simulink model "Aearial_Inspection_UAV_Simulation"  (R2023a)
settings: Solver=daessc  StartTime=0.0  StopTime=tf  MaxStep=0.1  MinStep=1e-30  RelTol=1e-4
values from neighbouring files (symbols this model uses):
  arm_start = 0    [InitScript.m]
  X = T*[x0;y0]    [line2circle.m]
undefined symbols (not defined in the file or in its folder): arm_end, DiscIntNeverNeededParam, F, is_gust_active, Light, MIL, Mode, Motor_data, params, Robotic_Arm_ASM_DataFile, Sensor_err, servo_specs, simple_env, stepper, Tm, wind_speed, xStack1, xStack2, Y, Z
libraries: sm_lib x399, nesl_utility x78, simulink x25, dspsrcs4 x16, simulink_extras x8, sharedtransform x7, aerolibwind2 x2, sharedutil x1
(part 2 of 12)

== system Aearial_Inspection_UAV_Simulation/UAV/Flange 1-1 ==
  PS-Simulink Converter : nesl_utility/PS-Simulink Converter  PhysicalDomain=network_engine_domain  SubClassName=ps_output  LeftPortType=input  RightPortType=output  PseudoPeriodic=off  Frequencies=[]  VectorFormat=1-D array  Unit=deg  AffineConversion=off
  Revolute : sm_lib/Joints/Revolute Joint  JointMode=Normal  SenseConstraintForce=off  SenseConstraintForceX=off  SenseConstraintForceY=off  SenseConstraintForceZ=off  SenseConstraintTorque=off  SenseConstraintTorqueX=off  SenseConstraintTorqueY=off  SenseConstraintTorqueZ=off  SenseTotalForce=off  SenseTotalForceX=off  SenseTotalForceY=off  SenseTotalForceZ=off  SenseTotalTorque=off  SenseTotalTorqueX=off  SenseTotalTorqueY=off  SenseTotalTorqueZ=off  CompositeWrenchDir=FollowerOnBase  CompositeWrenchFrame=BaseFrame  EquilibriumPosition=-360*2  EquilibriumPositionUnits=deg  SpringStiffness=1e-5  SpringStiffnessUnits=N*m/deg  DampingCoefficient=3e-6  DampingCoefficientUnits=N*m/(deg/s)  TorqueActuationMode=NoTorque  MotionActuationMode=ComputedMotion  SensePosition=on  SenseVelocity=off  SenseAcceleration=off  SenseTorqueForce=off  SenseLowerLimitTorqueForce=off  SenseUpperLimitTorqueForce=off  LowerLimitSpecify=on  LowerLimitBound=0  LowerLimitBoundUnits=deg  LowerLimitStiffness=1e-2  LowerLimitStiffnessUnits=N*m/deg  LowerLimitDamping=1  LowerLimitDampingUnits=N*m/(deg/s)  LowerLimitTransitionRegionWidth=0.1  LowerLimitTransitionRegionWidthUnits=deg  UpperLimitSpecify=on  UpperLimitBound=80  UpperLimitBoundUnits=deg  UpperLimitStiffness=1  UpperLimitStiffnessUnits=N*m/deg  UpperLimitDamping=1000  UpperLimitDampingUnits=N*m/(deg/s)  UpperLimitTransitionRegionWidth=0.1  UpperLimitTransitionRegionWidthUnits=deg  PositionTargetSpecify=on  PositionTargetPriority=Low  PositionTargetValue=10  PositionTargetValueUnits=deg  VelocityTargetSpecify=off  VelocityTargetPriority=High  VelocityTargetValue=0  VelocityTargetValueUnits=deg/s
  Transform : sm_lib/Frames and Transforms/Rigid Transform  TranslationMethod=Cartesian  TranslationStandardOffset=0  TranslationStandardOffsetUnits=m  TranslationStandardAxis=+Z  TranslationCartesianOffset=env.flange1_1.pos  TranslationCartesianOffsetUnits=m  TranslationROffset=0  TranslationROffsetUnits=m  TranslationZOffset=0  TranslationZOffsetUnits=m  TranslationThetaOffset=0  TranslationThetaOffsetUnits=deg  RotationMethod=RotationSequence  RotationAngleUnits=rad  RotationStandardAxis=+Z  RotationAngle=smiData.RigidTransform(3).angle  RotationArbitraryAxis=smiData.RigidTransform(3).axis  FollAlignAxisA=+X  BaseAlignAxisA=+Y  FollAlignAxisB=+Y  BaseAlignAxisB=+Z  RotationSequenceAxes=BaseAxes  RotationSequence=ZYX  RotationSequenceAngles=[90 -90 0]  RotationSequenceAnglesUnits=deg  RotationMatrix=[1 0 0; 0 1 0; 0 0 1]  Quaternion=[1 0 0 0]
  flange_1_RIGID : Subsystem
  flange_gate_1_RIGID : Subsystem
  Conn1 : PMIOPort  Side=Left
  Flange Door : PMIOPort  Port=2  Side=Right
  rot flange 1-1 : Outport
  wires:
  PS-Simulink Converter/1 -> rot flange 1-1/1
  connections:
  Conn1/RConn1 -- Transform/LConn1
  Transform/RConn1 -- flange_1_RIGID/LConn1
  Revolute/RConn1 -- flange_gate_1_RIGID/LConn1
  Revolute/LConn1 -- flange_1_RIGID/RConn1
  Flange Door/RConn1 -- flange_gate_1_RIGID/LConn2
  Revolute/RConn2 -- PS-Simulink Converter/LConn1

== system Aearial_Inspection_UAV_Simulation/UAV/Robotic Arm ==
  servos pos [6] : Inport
  Degrees to Radians : simulink_extras/Transformations/Degrees to Radians
  Demux : Demux  Outputs=6
  Gain : Gain  Gain=-1
  Gain2 : Gain  Gain=-1
  Mux : Mux  Inputs=6
  Robotic Arm and Servos : Subsystem
  Transport Delay : TransportDelay  DelayTime=0.001
  Transport Delay1 : TransportDelay  DelayTime=0.001
  ArmHolder : PMIOPort  Side=Left
  prob Geo : PMIOPort  Port=2  Side=Left
  prob head : PMIOPort  Port=3  Side=Left
  arms_real_rot_deg : Outport
  probHeadPos (disconnected) : Outport  Port=2
  probDiskPos : Outport  Port=3
  wires:
  Demux/5 -> Gain2/1
  Demux/6 -> Robotic Arm and Servos/6(w3)
  Transport Delay1/1 -> probDiskPos/1
  Degrees to Radians/1 -> Demux/1
  Transport Delay/1 -> arms_real_rot_deg/1
  Gain/1 -> Robotic Arm and Servos/1(a0)
  Robotic Arm and Servos/8(probDiskPos) -> Transport Delay1/1
  Robotic Arm and Servos/7(probHeadPos (disconnected)) -> probHeadPos (disconnected)/1
  Robotic Arm and Servos/6(w3_real) -> Mux/6
  Robotic Arm and Servos/4(w1_real) -> Mux/4
  Robotic Arm and Servos/5(w2_real) -> Mux/5
  Robotic Arm and Servos/2(a1_real) -> Mux/2
  Robotic Arm and Servos/3(a2_real) -> Mux/3
  Robotic Arm and Servos/1(a0_real) -> Mux/1
  Mux/1 -> Transport Delay/1
  servos pos [6]/1 -> Degrees to Radians/1
  Demux/4 -> Robotic Arm and Servos/4(w1)
  Gain2/1 -> Robotic Arm and Servos/5(w2)
  Demux/3 -> Robotic Arm and Servos/3(a2)
  Demux/1 -> Gain/1
  Demux/2 -> Robotic Arm and Servos/2(a1)
  connections:
  prob head/RConn1 -- Robotic Arm and Servos/LConn3
  prob Geo/RConn1 -- Robotic Arm and Servos/LConn2
  ArmHolder/RConn1 -- Robotic Arm and Servos/LConn1

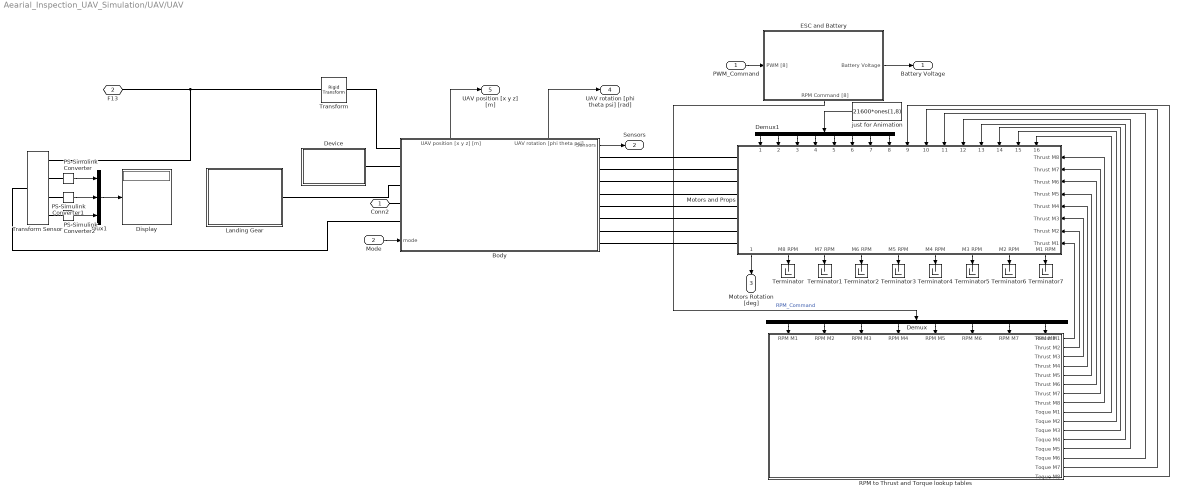
== system Aearial_Inspection_UAV_Simulation/UAV/UAV ==
  PWM_Command : Inport
  Mode : Inport  Port=2
  Body : Subsystem
      settings: PortSchema="{\"entries\":[{\"content\":{\"sides\":[{\"content\":{\"connectorIds\":[\"LConn1\",\"LConn2\",\"LConn3\",\"LConn4\",\"LConn5\",\"In1\"]},\"type\":\"ConnectorPlacement.EquallySpacedRectSide\",\"uuid\":\"8abbfab2-f266-443b-993d-92a00d5129d3\"},{\"content\":{\"connectorIds\":[\"Out1\",\"RConn1\",\"RConn2\",\"RConn3\",\"RConn4\",\"RConn5\",\"RConn6\",\"RConn7\",\"RConn8\"],\"side\":\"RIGHT\"},\"type\":\"ConnectorPlacement.EquallySpacedRectSide\",\"uuid\":\"d3862e7a-1f62-4fff-84ef-3f151d54fb23\"},{\"content\":{\"connectorIds\":[\"Out2\",\"Out3\"],\"side\":\"TOP\"},\"type\":\"ConnectorPlacement.EquallySpacedRectSide\",\"uuid\":\"186dc438-5235-44e9-8ffb-2a07ea9e8cef\"}]},\"type\":\"ConnectorPlacement.EquallySpacedConnector\",\"uuid\":\"6424af0a-0cb2-4ac3-b98a-3d9cf8166d6d\"}],\"packageUris\":[\"http://schema.mathworks.com/mf0/Connector/R2020b\"],\"version\":\"1.0\"}"
      mask Display: image('D:\MS_Control_Project\pictures\CH5\UAV.JPG'); % Use "Edit Image" on toolstrip to change.
  Demux : Demux  Outputs=8
  Demux1 : Demux  Outputs=8
  Device : Subsystem
      mask Display: image('D:\MS_Control_Project\pictures\CH3\test350.JPG'); % Use "Edit Image" on toolstrip to change.
  Display : Display
  ESC and Battery : Subsystem
      settings: PortSchema="{\"entries\":[{\"content\":{\"sides\":[{\"content\":{\"connectorIds\":[]},\"type\":\"ConnectorPlacement.EquallySpacedRectSide\",\"uuid\":\"711663de-8dcc-49e0-b3a9-e528dcc5693d\"},{\"content\":{\"connectorIds\":[\"Out1\"],\"side\":\"RIGHT\"},\"type\":\"ConnectorPlacement.EquallySpacedRectSide\",\"uuid\":\"6f86bd31-ad4a-448e-be8f-fb164a73c091\"},{\"content\":{\"connectorIds\":[\"In1\"],\"side\":\"TOP\"},\"type\":\"ConnectorPlacement.EquallySpacedRectSide\",\"uuid\":\"20362943-c19a-4854-b367-6ab35e814521\"},{\"content\":{\"connectorIds\":[\"Out2\"],\"side\":\"BOTTOM\"},\"type\":\"ConnectorPlacement.EquallySpacedRectSide\",\"uuid\":\"05de8953-dfce-4a54-9043-b5e6de62a3cd\"}]},\"type\":\"ConnectorPlacement.EquallySpacedConnector\",\"uuid\":\"7185b2e0-7de4-4151-8ca9-e57776bd11c7\"}],\"packageUris\":[\"http://schema.mathworks.com/mf0/Connector/R2020b\"],\"version\":\"1.0\"}"
  Landing Gear : Subsystem
  Motors and Props : Subsystem
      settings: PortSchema="{\"entries\":[{\"content\":{\"sides\":[{\"content\":{\"connectorIds\":[\"LConn1\",\"LConn2\",\"LConn3\",\"LConn4\",\"LConn5\",\"LConn6\",\"LConn7\",\"LConn8\"]},\"type\":\"ConnectorPlacement.EquallySpacedRectSide\",\"uuid\":\"df44c6ad-f38c-4e0a-a4d8-2c23b112f28a\"},{\"content\":{\"connectorIds\":[\"In17\",\"In18\",\"In19\",\"In20\",\"In21\",\"In22\",\"In23\",\"In24\"],\"side\":\"RIGHT\"},\"type\":\"ConnectorPlacement.EquallySpacedRectSide\",\"uuid\":\"523caf36-7a83-48a0-a73d-1fb2051ba00a\"},{\"content\":{\"connectorIds\":[\"In1\",\"In2\",\"In3\",\"In4\",\"In5\",\"In6\",\"In7\",\"In8\",\"In9\",\"In10\",\"In11\",\"In12\",\"In13\",\"In14\",\"In15\",\"In16\"],\"side\":\"TOP\"},\"type\":\"ConnectorPlacement.EquallySpacedRectSide\",\"uuid\":\"ed00d928-f4f1-4152-a592-487d88c7be46\"},{\"content\":{\"connectorIds\":[\"Out1\",\"Out2\",\"Out3\",\"Out4\",\"Out5\",\"Out6\",\"Out7\",\"Out8\",\"Out9\"],\"side\":\"BOTTOM\"},\"type\":\"ConnectorPlacement.EquallySpacedRectSide\",\"uuid\":\"181016b2-11c7-4594-b58c-8221d4cffb47\"}]},\"type\":\"ConnectorPlacement.EquallySpacedConnector\",\"uuid\":\"b878f0ff-a82a-4258-9edd-ea8bbdd36818\"}],\"packageUris\":[\"http://schema.mathworks.com/mf0/Connector/R2020b\"],\"version\":\"1.0\"}"
      mask Display: image('D:\MS_Control_Project\pictures\CH3\p60 with prop.JPG'); % Use "Edit Image" on toolstrip to change.
  Mux1 : Mux  Inputs=3
  PS-Simulink Converter : nesl_utility/PS-Simulink Converter  PhysicalDomain=network_engine_domain  SubClassName=ps_output  LeftPortType=input  RightPortType=output  PseudoPeriodic=off  Frequencies=[]  VectorFormat=1-D array  Unit=inherit  AffineConversion=off
  PS-Simulink Converter1 : nesl_utility/PS-Simulink Converter  PhysicalDomain=network_engine_domain  SubClassName=ps_output  LeftPortType=input  RightPortType=output  PseudoPeriodic=off  Frequencies=[]  VectorFormat=1-D array  Unit=inherit  AffineConversion=off
  PS-Simulink Converter2 : nesl_utility/PS-Simulink Converter  PhysicalDomain=network_engine_domain  SubClassName=ps_output  LeftPortType=input  RightPortType=output  PseudoPeriodic=off  Frequencies=[]  VectorFormat=1-D array  Unit=inherit  AffineConversion=off
  RPM to Thrust and Torque lookup tables : Subsystem
      settings: PortSchema="{\"entries\":[{\"content\":{\"sides\":[{\"content\":{\"connectorIds\":[]},\"type\":\"ConnectorPlacement.EquallySpacedRectSide\",\"uuid\":\"e225c0ad-404f-4beb-bd3c-0cf073c7c3b6\"},{\"content\":{\"connectorIds\":[\"Out1\",\"Out2\",\"Out3\",\"Out4\",\"Out5\",\"Out6\",\"Out7\",\"Out8\",\"Out9\",\"Out10\",\"Out11\",\"Out12\",\"Out13\",\"Out14\",\"Out15\",\"Out16\"],\"side\":\"RIGHT\"},\"type\":\"ConnectorPlacement.EquallySpacedRectSide\",\"uuid\":\"ade02e52-3795-4ae7-8485-9b36c688ef9f\"},{\"content\":{\"connectorIds\":[\"In1\",\"In2\",\"In3\",\"In4\",\"In5\",\"In6\",\"In7\",\"In8\"],\"side\":\"TOP\"},\"type\":\"ConnectorPlacement.EquallySpacedRectSide\",\"uuid\":\"a41127fa-8705-473b-8191-192aa5d830a9\"}]},\"type\":\"ConnectorPlacement.EquallySpacedConnector\",\"uuid\":\"d5038a5f-1241-42ee-bed9-472ac5262e65\"}],\"packageUris\":[\"http://schema.mathworks.com/mf0/Connector/R2020b\"],\"version\":\"1.0\"}"
  Terminator{,1..7} (8 alike) : Terminator
  Transform : sm_lib/Frames and Transforms/Rigid Transform  TranslationMethod=Cartesian  TranslationStandardOffset=0  TranslationStandardOffsetUnits=mm  TranslationStandardAxis=+Z  TranslationCartesianOffset=[-138 23.5 29.5]  TranslationCartesianOffsetUnits=mm  TranslationROffset=0  TranslationROffsetUnits=m  TranslationZOffset=0  TranslationZOffsetUnits=m  TranslationThetaOffset=0  TranslationThetaOffsetUnits=deg  RotationMethod=StandardAxis  RotationAngleUnits=deg  RotationStandardAxis=+Z  RotationAngle=-90  RotationArbitraryAxis=smiData.RigidTransform(37).axis  FollAlignAxisA=+X  BaseAlignAxisA=+Y  FollAlignAxisB=+Y  BaseAlignAxisB=+Z  RotationSequenceAxes=FollowerAxes  RotationSequence=XYX  RotationSequenceAngles=[0 0 0]  RotationSequenceAnglesUnits=deg  RotationMatrix=[1 0 0; 0 1 0; 0 0 1]  Quaternion=[1 0 0 0]
  Transform Sensor : sm_lib/Frames and Transforms/Transform Sensor  MeasurementFrame=Base  RotationSequence=XYX  SenseAngle=off  SenseAxis=off  SenseQ=off  SenseR=off  SenseRotationSequence=off  SenseOmegaX=off  SenseOmegaY=off  SenseOmegaZ=off  SenseQDot=off  SenseRDot=off  SenseRotationSequenceDot=off  SenseAlphaX=off  SenseAlphaY=off  SenseAlphaZ=off  SenseQDDot=off  SenseRDDot=off  SenseX=on  SenseY=on  SenseZ=on  SenseRad=off  SenseAzim=off  SenseDist=off  SenseInc=off  SenseXDot=off  SenseYDot=off  SenseZDot=off  SenseRadDot=off  SenseAzimDot=off  SenseDistDot=off  SenseIncDot=off  SenseXDDot=off  SenseYDDot=off  SenseZDDot=off  SenseRadDDot=off  SenseAzimDDot=off  SenseDistDDot=off  SenseIncDDot=off
  just for Animation : Constant  Value=21600*ones(1,8)
  Conn2 : PMIOPort  Side=Left
  F13 : PMIOPort  Port=2  Side=Left
  Battery Voltage : Outport
  Sensors : Outport  Port=2
  Motors Rotation [deg] : Outport  Port=3
  UAV rotation [phi theta psi] [rad] : Outport  Port=4
  UAV position [x y z] [m] : Outport  Port=5
  wires:
  PWM_Command/1 -> ESC and Battery/1(PWM [8])
  ESC and Battery/1(RPM Command [8]) -> Demux/1  "RPM_Command"
  RPM to Thrust and Torque lookup tables/1(Thrust M1) -> Motors and Props/24(Thrust M1)
  RPM to Thrust and Torque lookup tables/2(Thrust M2) -> Motors and Props/23(Thrust M2)
  RPM to Thrust and Torque lookup tables/3(Thrust M3) -> Motors and Props/22(Thrust M3)
  RPM to Thrust and Torque lookup tables/4(Thrust M4) -> Motors and Props/21(Thrust M4)
  RPM to Thrust and Torque lookup tables/5(Thrust M5) -> Motors and Props/20(Thrust M5)
  RPM to Thrust and Torque lookup tables/6(Thrust M6) -> Motors and Props/19(Thrust M6)
  RPM to Thrust and Torque lookup tables/7(Thrust M7) -> Motors and Props/18(Thrust M7)
  RPM to Thrust and Torque lookup tables/8(Thrust M8) -> Motors and Props/17(Thrust M8)
  RPM to Thrust and Torque lookup tables/9(Toque M1) -> Motors and Props/16(Torque M1)
  RPM to Thrust and Torque lookup tables/10(Toque M2) -> Motors and Props/15(Torque M2)
  RPM to Thrust and Torque lookup tables/11(Toque M3) -> Motors and Props/14(Torque M3)
  RPM to Thrust and Torque lookup tables/12(Toque M4) -> Motors and Props/13(Torque M4)
  RPM to Thrust and Torque lookup tables/13(Toque M5) -> Motors and Props/12(Torque M5)
  RPM to Thrust and Torque lookup tables/14(Toque M6) -> Motors and Props/11(Torque M6)
  RPM to Thrust and Torque lookup tables/15(Toque M7) -> Motors and Props/10(Torque M7)
  RPM to Thrust and Torque lookup tables/16(Toque M8) -> Motors and Props/9(Torque M8)
  ESC and Battery/2(Battery Voltage) -> Battery Voltage/1
  Body/1(Sensors) -> Sensors/1
  Motors and Props/1(Motors Rotation [deg]) -> Motors Rotation [deg]/1
  Body/3(UAV rotation [phi theta psi]) -> UAV rotation [phi theta psi] [rad]/1
  Body/2(UAV position [x y z] [m]) -> UAV position [x y z] [m]/1
  Demux/8 -> RPM to Thrust and Torque lookup tables/8(RPM M8)
  Demux/7 -> RPM to Thrust and Torque lookup tables/7(RPM M7)
  Demux/6 -> RPM to Thrust and Torque lookup tables/6(RPM M6)
  Demux/5 -> RPM to Thrust and Torque lookup tables/5(RPM M5)
  Demux/4 -> RPM to Thrust and Torque lookup tables/4(RPM M4)
  Demux/3 -> RPM to Thrust and Torque lookup tables/3(RPM M3)
  Demux/2 -> RPM to Thrust and Torque lookup tables/2(RPM M2)
  Demux/1 -> RPM to Thrust and Torque lookup tables/1(RPM M1)
  PS-Simulink Converter1/1 -> Mux1/2
  PS-Simulink Converter2/1 -> Mux1/3
  PS-Simulink Converter/1 -> Mux1/1
  Mux1/1 -> Display/1
  Demux1/1 -> Motors and Props/1(M1 RPM Command)
  Demux1/2 -> Motors and Props/2(M2 RPM Command)
  Demux1/3 -> Motors and Props/3(M3 RPM Command)
  Demux1/4 -> Motors and Props/4(M4 RPM Command)
  Demux1/5 -> Motors and Props/5(M5 RPM Command)
  Demux1/6 -> Motors and Props/6(M6 RPM Command)
  Demux1/7 -> Motors and Props/7(M7 RPM Command)
  Demux1/8 -> Motors and Props/8(M8 RPM Command)
  Motors and Props/2(M8 RPM) -> Terminator/1
  Motors and Props/3(M7 RPM) -> Terminator1/1
  Motors and Props/5(M5 RPM) -> Terminator3/1
  Motors and Props/4(M6 RPM) -> Terminator2/1
  Motors and Props/6(M4 RPM) -> Terminator4/1
  Motors and Props/7(M3 RPM) -> Terminator5/1
  Motors and Props/8(M2 RPM) -> Terminator6/1
  Motors and Props/9(M1 RPM) -> Terminator7/1
  just for Animation/1 -> Demux1/1
  Mode/1 -> Body/1(mode)
  connections:
  Device/LConn1 -- Body/LConn2
  Body/RConn5 -- Motors and Props/LConn5
  Body/RConn6 -- Motors and Props/LConn6
  Body/RConn3 -- Motors and Props/LConn3
  Body/RConn1 -- Motors and Props/LConn1
  Body/RConn7 -- Motors and Props/LConn7
  Body/LConn3 -- Landing Gear/LConn1
  Body/RConn4 -- Motors and Props/LConn4
  Body/RConn2 -- Motors and Props/LConn2
  Body/RConn8 -- Motors and Props/LConn8
  Conn2/RConn1 -- Body/LConn4
  Transform/RConn1 -- Transform Sensor/RConn1 -- F13/RConn1
  Transform/LConn1 -- Body/LConn1
  Transform Sensor/LConn1 -- Body/LConn5
  PS-Simulink Converter/LConn1 -- Transform Sensor/RConn2
  PS-Simulink Converter1/LConn1 -- Transform Sensor/RConn3
  PS-Simulink Converter2/LConn1 -- Transform Sensor/RConn4

== system Aearial_Inspection_UAV_Simulation/UAV/simple environment ==
  Rigid Transform : sm_lib/Frames and Transforms/Rigid Transform  TranslationMethod=Cartesian  TranslationStandardOffset=0  TranslationStandardOffsetUnits=m  TranslationStandardAxis=+Z  TranslationCartesianOffset=[simple_env.stack1_x simple_env.stack1_y -5.03]  TranslationCartesianOffsetUnits=m  TranslationROffset=0  TranslationROffsetUnits=m  TranslationZOffset=0  TranslationZOffsetUnits=m  TranslationThetaOffset=0  TranslationThetaOffsetUnits=deg  RotationMethod=RotationSequence  RotationAngleUnits=deg  RotationStandardAxis=+Z  RotationAngle=0.0  RotationArbitraryAxis=[0 0 1]  FollAlignAxisA=+X  BaseAlignAxisA=+Y  FollAlignAxisB=+Y  BaseAlignAxisB=+Z  RotationSequenceAxes=FollowerAxes  RotationSequence=ZYX  RotationSequenceAngles=[0 0 -90]  RotationSequenceAnglesUnits=deg  RotationMatrix=[1 0 0; 0 1 0; 0 0 1]  Quaternion=[1 0 0 0]
  Rigid Transform1 : sm_lib/Frames and Transforms/Rigid Transform  TranslationMethod=Cartesian  TranslationStandardOffset=0  TranslationStandardOffsetUnits=m  TranslationStandardAxis=+Z  TranslationCartesianOffset=[simple_env.stack2_x simple_env.stack2_y -5.03]  TranslationCartesianOffsetUnits=m  TranslationROffset=0  TranslationROffsetUnits=m  TranslationZOffset=0  TranslationZOffsetUnits=m  TranslationThetaOffset=0  TranslationThetaOffsetUnits=deg  RotationMethod=RotationSequence  RotationAngleUnits=deg  RotationStandardAxis=+Z  RotationAngle=0.0  RotationArbitraryAxis=[0 0 1]  FollAlignAxisA=+X  BaseAlignAxisA=+Y  FollAlignAxisB=+Y  BaseAlignAxisB=+Z  RotationSequenceAxes=FollowerAxes  RotationSequence=XYZ  RotationSequenceAngles=[-90 0 0]  RotationSequenceAnglesUnits=deg  RotationMatrix=[1 0 0; 0 1 0; 0 0 1]  Quaternion=[1 0 0 0]
  Rigid Transform2 : sm_lib/Frames and Transforms/Rigid Transform  TranslationMethod=Cartesian  TranslationStandardOffset=0  TranslationStandardOffsetUnits=m  TranslationStandardAxis=+Z  TranslationCartesianOffset=[0.7 0 21.2]  TranslationCartesianOffsetUnits=m  TranslationROffset=0  TranslationROffsetUnits=m  TranslationZOffset=0  TranslationZOffsetUnits=m  TranslationThetaOffset=0  TranslationThetaOffsetUnits=deg  RotationMethod=None  RotationAngleUnits=deg  RotationStandardAxis=+Z  RotationAngle=0.0  RotationArbitraryAxis=[0 0 1]  FollAlignAxisA=+X  BaseAlignAxisA=+Y  FollAlignAxisB=+Y  BaseAlignAxisB=+Z  RotationSequenceAxes=FollowerAxes  RotationSequence=XYX  RotationSequenceAngles=[0 0 0]  RotationSequenceAnglesUnits=deg  RotationMatrix=[1 0 0; 0 1 0; 0 0 1]  Quaternion=[1 0 0 0]
  Stack 1 : sm_lib/Body Elements/File Solid  ExtGeomFileName=D:\MS_Control_Project\Industrial_Chimneys_Aerial_Inspection_UAV\SolidWorks output\chimney\AssemChimney1.3M.SLDASM  UnitType=FromFile  ExtGeomFileUnits=m  StepReaderType=HEX  ExportConvexHullGeometry=off  InertiaType=CalculateFromGeometry  Mass=1  MassUnits=kg  CenterOfMass=[0 0 0]  CenterOfMassUnits=m  MomentsOfInertia=[1 1 1]  MomentsOfInertiaUnits=kg*m^2  ProductsOfInertia=[0 0 0]  ProductsOfInertiaUnits=kg*m^2  BasedOnType=Mass  Density=1000  DensityUnits=kg/m^3  DoExposeReferenceFrame=on  SerializedFrames=<Frames/>  GraphicType=FromGeometry  MarkerShape=Sphere  MarkerSize=10  GraphicVisPropType=SimpleVisualProperties  GraphicDiffuseColor=[0.5 0.5 0.5]  GraphicSpecularColor=[0.5 0.5 0.5 1.0]  GraphicAmbientColor=[0.15 0.15 0.15 1.0]  GraphicEmissiveColor=[0.0 0.0 0.0 1.0]  GraphicShininess=75  GraphicOpacity=1.0
  Stack 2 : sm_lib/Body Elements/File Solid  ExtGeomFileName=D:\MS_Control_Project\Industrial_Chimneys_Aerial_Inspection_UAV\SolidWorks output\chimney\AssemChimney1.3M.SLDASM  UnitType=FromFile  ExtGeomFileUnits=m  StepReaderType=HEX  ExportConvexHullGeometry=off  InertiaType=CalculateFromGeometry  Mass=1  MassUnits=kg  CenterOfMass=[0 0 0]  CenterOfMassUnits=m  MomentsOfInertia=[1 1 1]  MomentsOfInertiaUnits=kg*m^2  ProductsOfInertia=[0 0 0]  ProductsOfInertiaUnits=kg*m^2  BasedOnType=Mass  Density=1000  DensityUnits=kg/m^3  DoExposeReferenceFrame=on  SerializedFrames=<Frames/>  GraphicType=FromGeometry  MarkerShape=Sphere  MarkerSize=10  GraphicVisPropType=SimpleVisualProperties  GraphicDiffuseColor=[0.5 0.5 0.5]  GraphicSpecularColor=[0.5 0.5 0.5 1.0]  GraphicAmbientColor=[0.15 0.15 0.15 1.0]  GraphicEmissiveColor=[0.0 0.0 0.0 1.0]  GraphicShininess=75  GraphicOpacity=1.0
  ground : sm_lib/Body Elements/Brick Solid  GraphicAmbientColor=[0.15 0.15 0.15 1.0]  BasedOnType=Density  BrickDimensions=[100 100 .01]  BrickDimensionsUnits=m  CenterOfMass=[0 0 0]  CenterOfMassUnits=m  GraphicDiffuseColor=[0.0 0.2 0.2]  Density=1000  DensityUnits=kg/m^3  DoExposeReferenceFrame=on  GraphicEmissiveColor=[0.0 0.0 0.0 1.0]  ExportEntireGeometry=off  SerializedFrames=<Frames/>  MarkerShape=Sphere  MarkerSize=10  GraphicType=FromGeometry  InertiaType=CalculateFromGeometry  Mass=1  MassUnits=kg  MomentsOfInertia=[1 1 1]  MomentsOfInertiaUnits=kg*m^2  GraphicOpacity=1.0  ProductsOfInertia=[0 0 0]  ProductsOfInertiaUnits=kg*m^2  GraphicShininess=75  GraphicSpecularColor=[0.5 0.5 0.5 1.0]  GraphicVisPropType=SimpleVisualProperties
  Connection Port : PMIOPort  Side=Left
  connections:
  ground/RConn1 -- Rigid Transform/LConn1 -- Rigid Transform2/RConn1 -- Rigid Transform1/LConn1
  Rigid Transform/RConn1 -- Stack 1/RConn1
  Stack 2/RConn1 -- Rigid Transform1/RConn1
  Connection Port/RConn1 -- Rigid Transform2/LConn1

== system Aearial_Inspection_UAV_Simulation/Controller/Arm Controller/Arm and Wrist Inv-kinematics ==
  Mode : Inport
  desired prob pos [x,y,z] : Inport  Port=2
  desired prob orientation : Inport  Port=3
  UAV Attitude : Inport  Port=4
  ArmMode : Inport  Port=5
  servos_feedback : Inport  Port=6
  Enable : EnablePort
  Cast To Boolean : DataTypeConversion  OutDataTypeStr=boolean  SaturateOnIntegerOverflow=off  RndMeth=Floor
  Demux : Demux  Outputs=3
  Mux : Mux  Inputs=2
  wrist Controller : Subsystem
      settings: PortSchema="{\"entries\":[{\"content\":{\"sides\":[{\"content\":{\"connectorIds\":[\"In1\"]},\"type\":\"ConnectorPlacement.EquallySpacedRectSide\",\"uuid\":\"4502644e-1146-46b4-b27c-15c4c4ca9081\"},{\"content\":{\"connectorIds\":[\"Out1\"],\"side\":\"RIGHT\"},\"type\":\"ConnectorPlacement.EquallySpacedRectSide\",\"uuid\":\"e725cb62-69b1-43ce-93bd-7401d62be9c6\"},{\"content\":{\"connectorIds\":[],\"side\":\"TOP\"},\"type\":\"ConnectorPlacement.EquallySpacedRectSide\",\"uuid\":\"40e41791-3185-4118-be2e-ebc369a15a56\"},{\"content\":{\"connectorIds\":[\"In2\",\"In3\",\"In4\"],\"side\":\"BOTTOM\"},\"type\":\"ConnectorPlacement.EquallySpacedRectSide\",\"uuid\":\"ef83c226-9add-4636-876d-69359a98f6c3\"}]},\"type\":\"ConnectorPlacement.EquallySpacedConnector\",\"uuid\":\"a9971539-b7a2-4684-bb4b-bbd409d88a12\"}],\"packageUris\":[\"http://schema.mathworks.com/mf0/Connector/R2020b\"],\"version\":\"1.0\"}"
  َArm_Controller : MATLAB Function  TreatAsAtomicUnit=on
  servos pos [6] : Outport
  wires:
  desired prob orientation/1 -> wrist Controller/1(prob psi desired [deg])
  Demux/1 -> َArm_Controller/2(xd)
  Demux/3 -> َArm_Controller/4(zd)
  Demux/2 -> َArm_Controller/3(yd)
  wrist Controller/1(w1 w2 w3 [deg]) -> Mux/2
  Mux/1 -> servos pos [6]/1
  UAV Attitude/1 -> wrist Controller/2(UAV Attitude), َArm_Controller/5(UAV_Attitude)
  desired prob pos [x,y,z]/1 -> Demux/1
  Mode/1 -> َArm_Controller/1(Mode)
  ArmMode/1 -> Cast To Boolean/1
  Cast To Boolean/1 -> َArm_Controller/6(ArmMode), wrist Controller/4(Arm Mode)
  servos_feedback/1 -> wrist Controller/3(servo_feedback)
  َArm_Controller/1(Servo_Angles) -> Mux/1

== system Aearial_Inspection_UAV_Simulation/Controller/Arm Controller/Enabled Subsystem ==
  Enable : EnablePort
  Arm Senario 2 : MATLAB Function  TreatAsAtomicUnit=on
  Clock : Clock
  Servo pos [6] : Outport
  wires:
  Arm Senario 2/1(y) -> Servo pos [6]/1
  Clock/1 -> Arm Senario 2/1(t)

== system Aearial_Inspection_UAV_Simulation/Controller/Arm Controller/Subsystem ==
  In1 : Inport
  Cast To Double : DataTypeConversion  OutDataTypeStr=double  SaturateOnIntegerOverflow=off  RndMeth=Floor
  Constant : Constant  Value=[0 60 60 0 0 0]
  Product : Product
  Out1 : Outport
  wires:
  Constant/1 -> Product/2
  In1/1 -> Cast To Double/1
  Cast To Double/1 -> Product/1
  Product/1 -> Out1/1

== system Aearial_Inspection_UAV_Simulation/Controller/UAV Controller/      1 ==
  desired Attitude : Inport
  Attitude : Inport  Port=2
  "     " : Subsystem  mask{wphi=50, wpsi=50}
      mask prompts: wphi "phi and theta Channle freq"; wpsi "psi channel freq"
      mask init:
      | Bphi = zeros(2,1);
      | Bphi(end) = wphi^2;
      | 
      | Aphi = zeros(2);
      | Aphi(1,2) = 1;
      | Aphi(end,:) = [-wphi^2 -2*wphi];
      | 
      | 
      | 
      | Btheta = Bphi;
      | Atheta = Aphi;
      | 
      | 
      | 
      | Bpsi = zeros(2,1);
      | Bpsi(end) = wpsi^2;
      | 
      | Apsi = zeros(2);
      | Apsi(1,2) = 1;
      | Apsi(end,:) = [-wpsi^2 -2*wpsi];
      mask Display: disp("TD-EU2BAR")
  Gain : Gain  Gain=K  Multiplication=Matrix(K*u)
  Gain1 : Gain  Gain=C  Multiplication=Matrix(K*u)
  MATLAB Function : MATLAB Function  TreatAsAtomicUnit=on
  Product : Product  Multiplication=Matrix(*)
  Subsystem : Subsystem
  Sum : Sum  Inputs=|-+
  Sum1 : Sum  Inputs=|++
  "desired Angular rate [p_d, q_d, r_d]" : Outport
  wires:
  desired Attitude/1 -> Sum/2, "     "/1(phi_d theta_d psi_d)
  Sum/1 -> MATLAB Function/1(Err_of_Atti), Gain/1
  "     "/1("[phi_d, phi_d_dot] [theta_d, theta_d_dot] [psi_d, psi_d_dot]") -> Gain1/1
  Gain/1 -> Sum1/1
  Gain1/1 -> Sum1/2
  Product/1 -> MATLAB Function/2(u)
  Attitude/1 -> Subsystem/1(In1), Sum/1
  Sum1/1 -> Product/2
  Subsystem/1(Matrix) -> Product/1
  MATLAB Function/1(y) -> "desired Angular rate [p_d, q_d, r_d]"/1

== system Aearial_Inspection_UAV_Simulation/Controller/UAV Controller/     1 ==
  "[xd, yd]" : Inport
  Demux : Demux  Outputs=2
  Gain : Gain  Gain=By  Multiplication=Matrix(K*u)
  Gain1 : Gain  Gain=Ay  Multiplication=Matrix(K*u)
  Gain2 : Gain  Gain=Bx  Multiplication=Matrix(K*u)
  Gain3 : Gain  Gain=Ax  Multiplication=Matrix(K*u)
  Integrator : Integrator  InitialCondition=zeros(3,1)
  Integrator1 : Integrator
  Mux : Mux  Inputs=2
  Sum : Sum  Inputs=|++
  Sum1 : Sum  Inputs=|++
  "[xd, xd_dot, xd_2dot] [yd, yd_dot, yd_2dot]" : Outport
  wires:
  "[xd, yd]"/1 -> Demux/1
  Gain/1 -> Sum/1
  Sum/1 -> Integrator/1
  Gain1/1 -> Sum/2
  Integrator/1 -> Gain1/1, Mux/2  "[yd, yd_dot, yd_2dot]"
  Mux/1 -> "[xd, xd_dot, xd_2dot] [yd, yd_dot, yd_2dot]"/1
  Integrator1/1 -> Gain3/1, Mux/1  "[xd, xd_dot, xd_2dot]"
  Gain3/1 -> Sum1/2
  Sum1/1 -> Integrator1/1
  Gain2/1 -> Sum1/1
  Demux/1 -> Gain2/1  "xd"
  Demux/2 -> Gain/1  "yd"

== system Aearial_Inspection_UAV_Simulation/Controller/UAV Controller/C-AAC  ==
  desired Atti : Inport
  x_hat : Inport  Port=2
  desired Altitiude : Inport  Port=3
  C-Alt : MATLAB Function  TreatAsAtomicUnit=on
  C-Atti : MATLAB Function  TreatAsAtomicUnit=on
  Constant : Constant  Value=wc_Alt
  Constant1 : Constant  Value=wp
  Constant2 : Constant  Value=wq
  Constant3 : Constant  Value=wr
  Gain : Gain
  Gain1 : Gain  Gain=params.M
  Gain2 : Gain  Gain=params.I.*[1 0 1;0 1 0;1 0 1]  Multiplication=Matrix(K*u)
  Mux : Mux  Inputs=2
  Signal router : Subsystem
      mask Display: disp("Signal router")
  Sum : Sum  Inputs=|+-
  u : Outport
  wires:
  Gain2/1 -> Mux/2
  C-Alt/1(u) -> Gain1/1
  Signal router/2(V-Alt) -> C-Alt/2(v_Alt)
  Gain1/1 -> Mux/1
  C-Atti/1(u) -> Gain2/1
  Signal router/1(Error-Alt) -> C-Alt/1(e_Alt)
  x_hat/1 -> Signal router/2(x_hat)
  Gain/1 -> u/1
  Sum/1 -> Gain/1
  Signal router/3(Error-Atti) -> C-Atti/1(e)
  Mux/1 -> Sum/1
  Signal router/4("desturbance ") -> Sum/2
  Constant/1 -> C-Alt/3(w_alt)
  Constant1/1 -> C-Atti/2(wp)
  Constant2/1 -> C-Atti/3(wq)
  Constant3/1 -> C-Atti/4(wr)
  desired Altitiude/1 -> Signal router/3(desired Alt)
  desired Atti/1 -> Signal router/1(desired Atti)

== system Aearial_Inspection_UAV_Simulation/Controller/UAV Controller/C-PC ==
  ref : Inport
  x_hat : Inport  Port=2
  C-Alt : MATLAB Function  TreatAsAtomicUnit=on
  Constant : Constant  Value=wc_x
  Gain : Gain
  Saturation : Saturate  UpperLimit=tand(20)*9.81  LowerLimit=-tand(20)*9.81  ZeroCross=off
  Scope : Scope  NumInputPorts=2
  Signal router : Subsystem
      mask Display: disp("Signal router")
  Sum : Sum  Inputs=|+-
  u : Outport
  wires:
  Signal router/1(Error-Pos) -> C-Alt/1(e_Pos)
  ref/1 -> Signal router/1(refs)
  Signal router/3(V-Pos) -> C-Alt/3(v_Pos)
  Saturation/1 -> Gain/1
  Gain/1 -> u/1
  x_hat/1 -> Signal router/2(x_hat)
  C-Alt/1(u) -> Scope/1, Sum/1
  Signal router/4("desturbance ") -> Scope/2, Sum/2
  Signal router/2(Vd) -> C-Alt/2(vd)
  Constant/1 -> C-Alt/4(wc_x)
  Sum/1 -> Saturation/1

== system Aearial_Inspection_UAV_Simulation/Controller/UAV Controller/ESO-AAC ==
  u : Inport  PortDimensions=4
  Angular Rate [p,q,r] : Inport  Port=2  PortDimensions=3
  "[Alt, Climb rate]" : Inport  Port=3  PortDimensions=2
  Gain : Gain  Gain=A  Multiplication=Matrix(K*u)
  Gain1 : Gain  Gain=L  Multiplication=Matrix(K*u)
  Gain2 : Gain  Gain=C  Multiplication=Matrix(K*u)
  Gain3 : Gain  Gain=B  Multiplication=Matrix(K*u)
  Integrator : Integrator
  Mux : Mux  Inputs=2
  Mux1 : Mux  Inputs=2
  Selector : Selector  InputPortWidth=9  IndexOptions=Index vector (dialog)  Indices=6:9  OutputSizes=1
  Sum : Sum  Inputs=|++
  Sum1 : Sum  Inputs=|++
  Sum2 : Sum  Inputs=-+|
  x_hat : Outport
  wires:
  Sum2/1 -> Gain1/1
  Sum1/1 -> Sum/2
  Gain/1 -> Sum1/2
  Mux/1 -> Mux1/1, Sum2/2
  Gain2/1 -> Sum2/1
  Sum/1 -> Integrator/1
  Gain1/1 -> Sum1/1
  Integrator/1 -> Gain/1, Gain2/1, Selector/1
  Gain3/1 -> Sum/1
  Angular Rate [p,q,r]/1 -> Mux/2
  "[Alt, Climb rate]"/1 -> Mux/1
  u/1 -> Gain3/1
  Selector/1 -> Mux1/2
  Mux1/1 -> x_hat/1

== system Aearial_Inspection_UAV_Simulation/Controller/UAV Controller/ESO-PC ==
  u : Inport  PortDimensions=2
  y : Inport  Port=2  PortDimensions=4
  Gain : Gain  Gain=A  Multiplication=Matrix(K*u)
  Gain1 : Gain  Gain=L  Multiplication=Matrix(K*u)
  Gain2 : Gain  Gain=C  Multiplication=Matrix(K*u)
  Gain3 : Gain  Gain=B  Multiplication=Matrix(K*u)
  Integrator : Integrator  InitialCondition=[params.pos0(1) 0 params.pos0(2) 0 0 0]
  Mux1 : Mux  Inputs=2
  Selector : Selector  InputPortWidth=6  IndexOptions=Index vector (dialog)  Indices=5:6  OutputSizes=1
  Sum : Sum  Inputs=|++
  Sum1 : Sum  Inputs=|++
  Sum2 : Sum  Inputs=-+|
  x_hat : Outport  PortDimensions=6
  wires:
  Sum/1 -> Integrator/1
  Integrator/1 -> Selector/1, Gain2/1, Gain/1
  Gain/1 -> Sum1/2
  Sum1/1 -> Sum/2
  Gain1/1 -> Sum1/1
  y/1 -> Sum2/2, Mux1/1
  Gain2/1 -> Sum2/1
  Sum2/1 -> Gain1/1
  Gain3/1 -> Sum/1
  u/1 -> Gain3/1
  Mux1/1 -> x_hat/1
  Selector/1 -> Mux1/2

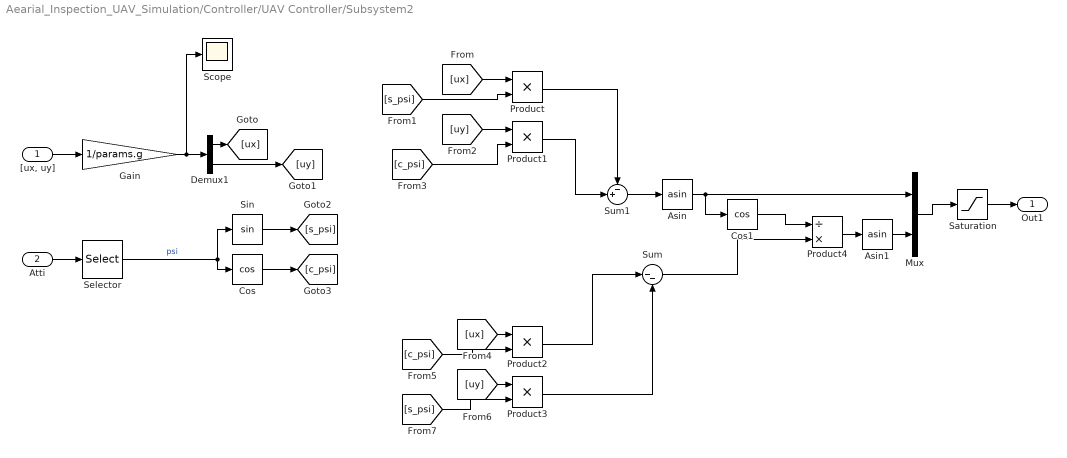
== system Aearial_Inspection_UAV_Simulation/Controller/UAV Controller/Subsystem2 ==
  "[ux, uy]" : Inport
  Atti : Inport  Port=2
  Asin : Trigonometry  Operator=asin
  Asin1 : Trigonometry  Operator=asin
  Cos : Trigonometry  Operator=cos
  Cos1 : Trigonometry  Operator=cos
  Demux1 : Demux  Outputs=2
  Gain : Gain  Gain=1/params.g
  Mux : Mux  Inputs=2
  Product{,1..3} (4 alike) : Product
  Product4 : Product  Inputs=/*
  Saturation : Saturate  UpperLimit=20*pi/180  LowerLimit=-20*pi/180
  Scope : Scope
  Selector : Selector  InputPortWidth=3  IndexOptions=Index vector (dialog)  Indices=3  OutputSizes=1
  Sin : Trigonometry
  Sum : Sum  Inputs=|--
  Sum1 : Sum  Inputs=-+|
  Out1 : Outport
  wires:
  Atti/1 -> Selector/1
  "[ux, uy]"/1 -> Gain/1
  Saturation/1 -> Out1/1
  Mux/1 -> Saturation/1
  Demux1/1 -> [ux]
  Demux1/2 -> [uy]
  Sin/1 -> [s_psi]
  Cos/1 -> [c_psi]
  Sum1/1 -> Asin/1
  Sum/1 -> Product4/2
  [ux] -> Product/1
  [s_psi] -> Product/2
  [uy] -> Product1/1
  [c_psi] -> Product1/2
  Product/1 -> Sum1/1
  Product1/1 -> Sum1/2
  [ux] -> Product2/1
  [c_psi] -> Product2/2
  [uy] -> Product3/1
  [s_psi] -> Product3/2
  Product2/1 -> Sum/1
  Product3/1 -> Sum/2
  Asin1/1 -> Mux/2
  Asin/1 -> Cos1/1, Mux/1
  Gain/1 -> Scope/1, Demux1/1
  Product4/1 -> Asin1/1
  Cos1/1 -> Product4/1
  Selector/1 -> Cos/1, Sin/1  "psi"

== system Aearial_Inspection_UAV_Simulation/Controller/UAV Controller/Subsystem3 ==
  Atti : Inport
  Constant : Constant  Value=[0 0 -9.81]
  Product : Product  Multiplication=Matrix(*)
  Rotation Angles to Direction Cosine Matrix : sharedtransform/Rotation Angles to Direction Cosine Matrix  rotationOrder=ZYX  aMode=aMode
  Selector : Selector  InputPortWidth=3  IndexOptions=Index vector (dialog)  Indices=[3 2 1]  OutputSizes=1
  Selector1 : Selector  InputPortWidth=3  IndexOptions=Index vector (dialog)  Indices=[1 2]  OutputSizes=1
  Transpose : Math  Operator=transpose
  Out1 : Outport
  wires:
  Atti/1 -> Selector/1
  Selector/1 -> Rotation Angles to Direction Cosine Matrix/1
  Rotation Angles to Direction Cosine Matrix/1 -> Transpose/1
  Product/1 -> Selector1/1
  Selector1/1 -> Out1/1
  Constant/1 -> Product/2
  Transpose/1 -> Product/1

== system Aearial_Inspection_UAV_Simulation/GPS-INS/GPS/Subsystem ==
  real Position data : Inport
  Gain : Gain  Gain=Sensor_err.gps.noise_Amp(1)
  Gain1 : Gain  Gain=Sensor_err.gps.noise_Amp(2)
  Gain2 : Gain  Gain=Sensor_err.gps.noise_Amp(3)
  Mux : Mux  Inputs=3
  Product : Product
  Product1 : Product
  Product2 : Product
  Random Source : dspsrcs4/Random Source  SrcType=Uniform  NormMethod=Ziggurat  CltLength=12  MinVal=0  MaxVal=1  MeanVal=0  VarVal=1  RepMode=Not repeatable  rawSeed=1  IsInherit=off  SampMode=Discrete  SampTime=1  SampFrame=1  DataType=Double  OutComplex=Real  OutputFrames=off
  Random Source1 : dspsrcs4/Random Source  SrcType=Uniform  NormMethod=Ziggurat  CltLength=12  MinVal=0  MaxVal=1  MeanVal=0  VarVal=1  RepMode=Not repeatable  rawSeed=1  IsInherit=off  SampMode=Discrete  SampTime=1  SampFrame=1  DataType=Double  OutComplex=Real  OutputFrames=off
  Random Source2 : dspsrcs4/Random Source  SrcType=Uniform  NormMethod=Ziggurat  CltLength=12  MinVal=0  MaxVal=1  MeanVal=0  VarVal=1  RepMode=Not repeatable  rawSeed=1  IsInherit=off  SampMode=Discrete  SampTime=1  SampFrame=1  DataType=Double  OutComplex=Real  OutputFrames=off
  Sine Wave : Sin  Frequency=2*pi*Sensor_err.gps.freqs_x  SampleTime=0
  Sine Wave1 : Sin  Frequency=2*pi*Sensor_err.gps.freqs_y  SampleTime=0
  Sine Wave2 : Sin  Frequency=2*pi*Sensor_err.gps.freqs_z  SampleTime=0
  Sum : Sum  Inputs=3
  Sum of Elements : Sum  Inputs=+
  Sum of Elements1 : Sum  Inputs=+
  Sum of Elements2 : Sum  Inputs=+
  gps bias : Constant  Value=Sensor_err.gps.bias
  gps output : Outport
  wires:
  Sum of Elements2/1 -> Gain2/1
  gps bias/1 -> Sum/3
  Sum of Elements1/1 -> Gain1/1
  Sum of Elements/1 -> Gain/1
  Sine Wave/1 -> Sum of Elements/1
  real Position data/1 -> Sum/2
  Sum/1 -> gps output/1
  Sine Wave2/1 -> Sum of Elements2/1
  Sine Wave1/1 -> Sum of Elements1/1
  Gain/1 -> Product/2
  Product1/1 -> Mux/2
  Mux/1 -> Sum/1
  Gain2/1 -> Product2/2
  Random Source2/1 -> Product2/1
  Product2/1 -> Mux/3
  Random Source1/1 -> Product1/1
  Gain1/1 -> Product1/2
  Product/1 -> Mux/1
  Random Source/1 -> Product/1

== system Aearial_Inspection_UAV_Simulation/GPS-INS/IMU/Acc ==
  real acc data : Inport
  Gain : Gain  Gain=Sensor_err.ax.noise_Amp
  Gain1 : Gain  Gain=Sensor_err.ay.noise_Amp
  Gain2 : Gain  Gain=Sensor_err.az.noise_Amp
  Mux1 : Mux  Inputs=3
  Product : Product
  Product1 : Product
  Product2 : Product
  Random Source : dspsrcs4/Random Source  SrcType=Uniform  NormMethod=Ziggurat  CltLength=12  MinVal=0  MaxVal=1  MeanVal=0  VarVal=1  RepMode=Not repeatable  rawSeed=1  IsInherit=off  SampMode=Continuous  SampTime=1  SampFrame=1  DataType=Double  OutComplex=Real  OutputFrames=off
  Random Source1 : dspsrcs4/Random Source  SrcType=Uniform  NormMethod=Ziggurat  CltLength=12  MinVal=0  MaxVal=1  MeanVal=0  VarVal=1  RepMode=Not repeatable  rawSeed=1  IsInherit=off  SampMode=Continuous  SampTime=1  SampFrame=1  DataType=Double  OutComplex=Real  OutputFrames=off
  Random Source2 : dspsrcs4/Random Source  SrcType=Uniform  NormMethod=Ziggurat  CltLength=12  MinVal=0  MaxVal=1  MeanVal=0  VarVal=1  RepMode=Not repeatable  rawSeed=1  IsInherit=off  SampMode=Continuous  SampTime=1  SampFrame=1  DataType=Double  OutComplex=Real  OutputFrames=off
  Sine Wave : Sin  Frequency=2*pi*Sensor_err.ax.freqs  SampleTime=0
  Sine Wave1 : Sin  Frequency=2*pi*Sensor_err.ay.freqs  SampleTime=0
  Sine Wave2 : Sin  Frequency=2*pi*Sensor_err.az.freqs  SampleTime=0
  Sum : Sum  Inputs=3
  Sum of Elements : Sum  Inputs=+
  Sum of Elements1 : Sum  Inputs=+
  Sum of Elements2 : Sum  Inputs=+
  acc bias : Constant  Value=[Sensor_err.ax.bias Sensor_err.ay.bias Sensor_err.az.bias]
  acc output : Outport
  wires:
  Sine Wave1/1 -> Sum of Elements1/1
  Sine Wave2/1 -> Sum of Elements2/1
  Sum/1 -> acc output/1
  real acc data/1 -> Sum/2
  Sine Wave/1 -> Sum of Elements/1
  Sum of Elements/1 -> Gain/1
  Sum of Elements1/1 -> Gain1/1
  Gain2/1 -> Product2/2
  acc bias/1 -> Sum/3
  Sum of Elements2/1 -> Gain2/1
  Gain1/1 -> Product1/2
  Gain/1 -> Product/2
  Product1/1 -> Mux1/2
  Mux1/1 -> Sum/1
  Random Source2/1 -> Product2/1
  Product2/1 -> Mux1/3
  Random Source1/1 -> Product1/1
  Product/1 -> Mux1/1
  Random Source/1 -> Product/1

== system Aearial_Inspection_UAV_Simulation/GPS-INS/IMU/Mag ==
  real mag data : Inport
  Gain2 : Gain  Gain=Sensor_err.mag.noise_Amp
  Product : Product
  Random Source : dspsrcs4/Random Source  SrcType=Uniform  NormMethod=Ziggurat  CltLength=12  MinVal=0  MaxVal=1  MeanVal=0  VarVal=1  RepMode=Not repeatable  rawSeed=1  IsInherit=off  SampMode=Continuous  SampTime=1  SampFrame=1  DataType=Double  OutComplex=Real  OutputFrames=off
  Sine Wave2 : Sin  Frequency=2*pi*Sensor_err.mag.freqs  SampleTime=0
  Sum : Sum  Inputs=3
  Sum of Elements2 : Sum  Inputs=+
  mag bias : Constant  Value=Sensor_err.mag.bias
  mag output : Outport
  wires:
  Sum of Elements2/1 -> Gain2/1
  mag bias/1 -> Sum/3
  real mag data/1 -> Sum/2
  Sum/1 -> mag output/1
  Sine Wave2/1 -> Sum of Elements2/1
  Gain2/1 -> Product/2
  Random Source/1 -> Product/1
  Product/1 -> Sum/1

== system Aearial_Inspection_UAV_Simulation/GPS-INS/IMU/Rotation ==
  real rotation data : Inport
  Gain : Gain  Gain=Sensor_err.ax.noise_Amp
  Gain1 : Gain  Gain=Sensor_err.ay.noise_Amp
  Gain2 : Gain  Gain=Sensor_err.az.noise_Amp
  Mux : Mux  Inputs=3
  Product : Product
  Product1 : Product
  Product2 : Product
  Random Source : dspsrcs4/Random Source  Commented=on  SrcType=Uniform  NormMethod=Ziggurat  CltLength=12  MinVal=0  MaxVal=1  MeanVal=0  VarVal=1  RepMode=Not repeatable  rawSeed=1  IsInherit=off  SampMode=Continuous  SampTime=1  SampFrame=1  DataType=Double  OutComplex=Real  OutputFrames=off
  Random Source1 : dspsrcs4/Random Source  Commented=on  SrcType=Uniform  NormMethod=Ziggurat  CltLength=12  MinVal=0  MaxVal=1  MeanVal=0  VarVal=1  RepMode=Not repeatable  rawSeed=1  IsInherit=off  SampMode=Continuous  SampTime=1  SampFrame=1  DataType=Double  OutComplex=Real  OutputFrames=off
  Random Source2 : dspsrcs4/Random Source  Commented=on  SrcType=Uniform  NormMethod=Ziggurat  CltLength=12  MinVal=0  MaxVal=1  MeanVal=0  VarVal=1  RepMode=Not repeatable  rawSeed=1  IsInherit=off  SampMode=Continuous  SampTime=1  SampFrame=1  DataType=Double  OutComplex=Real  OutputFrames=off
  Sine Wave : Sin  Frequency=2*pi*Sensor_err.rx.freqs  SampleTime=0
  Sine Wave1 : Sin  Frequency=2*pi*Sensor_err.ry.freqs  SampleTime=0
  Sine Wave2 : Sin  Frequency=2*pi*Sensor_err.rz.freqs  SampleTime=0
  Sum : Sum  Inputs=3
  Sum of Elements : Sum  Inputs=+
  Sum of Elements1 : Sum  Inputs=+
  Sum of Elements2 : Sum  Inputs=+
  To Workspace : ToWorkspace  VariableName=atti  SaveFormat=Timeseries  SampleTime=-1
  angle jump correction : Subsystem
  rotation bias : Constant  Value=[Sensor_err.rx.bias Sensor_err.ry.bias Sensor_err.rz.bias]
  rotation : Outport
  wires:
  Gain/1 -> Product/2
  Gain1/1 -> Product1/2
  Sum of Elements2/1 -> Gain2/1
  rotation bias/1 -> Sum/3
  Gain2/1 -> Product2/2
  Sum of Elements1/1 -> Gain1/1
  Sum of Elements/1 -> Gain/1
  Sine Wave/1 -> Sum of Elements/1
  Sum/1 -> rotation/1
  Sine Wave2/1 -> Sum of Elements2/1
  Sine Wave1/1 -> Sum of Elements1/1
  Mux/1 -> Sum/1
  Random Source/1 -> Product/1
  Product1/1 -> Mux/2
  Product/1 -> Mux/1
  Product2/1 -> Mux/3
  Random Source1/1 -> Product1/1
  Random Source2/1 -> Product2/1
  real rotation data/1 -> angle jump correction/1(u)
  angle jump correction/1(y) -> To Workspace/1, Sum/2

== system Aearial_Inspection_UAV_Simulation/GPS-INS/IMU/Vel Imu ==
  real acc data : Inport
  Gain : Gain  Gain=Sensor_err.vel.noise_Amp(1)
  Gain1 : Gain  Gain=Sensor_err.vel.noise_Amp(2)
  Gain2 : Gain  Gain=Sensor_err.vel.noise_Amp(3)
  Mux1 : Mux  Inputs=3
  Product : Product
  Product1 : Product
  Product2 : Product
  Random Source : dspsrcs4/Random Source  Commented=on  SrcType=Uniform  NormMethod=Ziggurat  CltLength=12  MinVal=0  MaxVal=1  MeanVal=0  VarVal=1  RepMode=Not repeatable  rawSeed=1  IsInherit=off  SampMode=Continuous  SampTime=1  SampFrame=1  DataType=Double  OutComplex=Real  OutputFrames=off
  Random Source1 : dspsrcs4/Random Source  Commented=on  SrcType=Uniform  NormMethod=Ziggurat  CltLength=12  MinVal=0  MaxVal=1  MeanVal=0  VarVal=1  RepMode=Not repeatable  rawSeed=1  IsInherit=off  SampMode=Continuous  SampTime=1  SampFrame=1  DataType=Double  OutComplex=Real  OutputFrames=off
  Random Source2 : dspsrcs4/Random Source  Commented=on  SrcType=Uniform  NormMethod=Ziggurat  CltLength=12  MinVal=0  MaxVal=1  MeanVal=0  VarVal=1  RepMode=Not repeatable  rawSeed=1  IsInherit=off  SampMode=Continuous  SampTime=1  SampFrame=1  DataType=Double  OutComplex=Real  OutputFrames=off
  Sine Wave : Sin  Frequency=2*pi*Sensor_err.vel.freqs_x  SampleTime=0
  Sine Wave1 : Sin  Frequency=2*pi*Sensor_err.vel.freqs_y  SampleTime=0
  Sine Wave2 : Sin  Frequency=2*pi*Sensor_err.vel.freqs_z  SampleTime=0
  Sum : Sum  Inputs=3
  Sum of Elements : Sum  Inputs=+
  Sum of Elements1 : Sum  Inputs=+
  Sum of Elements2 : Sum  Inputs=+
  acc bias : Constant  Value=Sensor_err.vel.bias
  acc output : Outport
  wires:
  Random Source/1 -> Product/1
  Product/1 -> Mux1/1
  Random Source1/1 -> Product1/1
  Product2/1 -> Mux1/3
  Random Source2/1 -> Product2/1
  Mux1/1 -> Sum/1
  Product1/1 -> Mux1/2
  Gain/1 -> Product/2
  Gain1/1 -> Product1/2
  Sum of Elements2/1 -> Gain2/1
  acc bias/1 -> Sum/3
  Gain2/1 -> Product2/2
  Sum of Elements1/1 -> Gain1/1
  Sum of Elements/1 -> Gain/1
  Sine Wave/1 -> Sum of Elements/1
  real acc data/1 -> Sum/2
  Sum/1 -> acc output/1
  Sine Wave2/1 -> Sum of Elements2/1
  Sine Wave1/1 -> Sum of Elements1/1

== system Aearial_Inspection_UAV_Simulation/GPS-INS/IMU/gyro ==
  real gyro data : Inport
  Gain : Gain  Gain=Sensor_err.gx.noise_Amp
  Gain1 : Gain  Gain=Sensor_err.gy.noise_Amp
  Gain2 : Gain  Gain=Sensor_err.gz.noise_Amp
  Mux : Mux  Inputs=3
  Product : Product
  Product1 : Product
  Product2 : Product
  Random Source : dspsrcs4/Random Source  Commented=on  SrcType=Uniform  NormMethod=Ziggurat  CltLength=12  MinVal=0  MaxVal=1  MeanVal=0  VarVal=1  RepMode=Not repeatable  rawSeed=1  IsInherit=off  SampMode=Continuous  SampTime=1  SampFrame=1  DataType=Double  OutComplex=Real  OutputFrames=off
  Random Source1 : dspsrcs4/Random Source  Commented=on  SrcType=Uniform  NormMethod=Ziggurat  CltLength=12  MinVal=0  MaxVal=1  MeanVal=0  VarVal=1  RepMode=Not repeatable  rawSeed=1  IsInherit=off  SampMode=Continuous  SampTime=1  SampFrame=1  DataType=Double  OutComplex=Real  OutputFrames=off
  Random Source2 : dspsrcs4/Random Source  Commented=on  SrcType=Uniform  NormMethod=Ziggurat  CltLength=12  MinVal=0  MaxVal=1  MeanVal=0  VarVal=1  RepMode=Not repeatable  rawSeed=1  IsInherit=off  SampMode=Continuous  SampTime=1  SampFrame=1  DataType=Double  OutComplex=Real  OutputFrames=off
  Sine Wave : Sin  Frequency=2*pi*Sensor_err.gx.freqs  SampleTime=0
  Sine Wave1 : Sin  Frequency=2*pi*Sensor_err.gy.freqs  SampleTime=0
  Sine Wave2 : Sin  Frequency=2*pi*Sensor_err.gz.freqs  SampleTime=0
  Sum : Sum  Inputs=3
  Sum of Elements : Sum  Inputs=+
  Sum of Elements1 : Sum  Inputs=+
  Sum of Elements2 : Sum  Inputs=+
  gyro bias : Constant  Value=[Sensor_err.gx.bias Sensor_err.gy.bias Sensor_err.gz.bias]
  Gyro output : Outport
  wires:
  Sum of Elements2/1 -> Gain2/1
  gyro bias/1 -> Sum/3
  Sum of Elements1/1 -> Gain1/1
  Sum of Elements/1 -> Gain/1
  Sine Wave/1 -> Sum of Elements/1
  real gyro data/1 -> Sum/2
  Sum/1 -> Gyro output/1
  Sine Wave2/1 -> Sum of Elements2/1
  Sine Wave1/1 -> Sum of Elements1/1
  Gain/1 -> Product/2
  Product1/1 -> Mux/2
  Mux/1 -> Sum/1
  Gain2/1 -> Product2/2
  Random Source2/1 -> Product2/1
  Product2/1 -> Mux/3
  Random Source1/1 -> Product1/1
  Gain1/1 -> Product1/2
  Product/1 -> Mux/1
  Random Source/1 -> Product/1

== system Aearial_Inspection_UAV_Simulation/Path Palnner/Arm Guid/Guidance Gate ==
  Sen1 pos : Inport
  psi sen 1 : Inport  Port=2
  Manual psi : Inport  Port=3
  Manual pos : Inport  Port=4
  psi sen 4 : Inport  Port=5
  pos Sen 4 : Inport  Port=6
  psi sen 5 : Inport  Port=7
  pos Sen 5 : Inport  Port=8
  pos Sen 2 : Inport  Port=9
  psi sen 2 : Inport  Port=10
  pos Sen 3 : Inport  Port=11
  psi sen 3 : Inport  Port=12
  Constant : Constant  Value=[0 0 0]
  Constant1 : Constant  Value=[0 0 0]
  Selector : Selector  InputPortWidth=3  IndexOptions=Index vector (dialog)  Indices=3  OutputSizes=1
  Sum{,1..2,5} (4 alike) : Sum  Inputs=3
  Sum{3..4,6..7} (4 alike) : Sum  Inputs=|++
  desired position : Outport
  desired Heading : Outport  Port=2
  wires:
  Manual pos/1 -> Sum/2
  Sen1 pos/1 -> Sum/3
  Manual psi/1 -> Sum1/2
  psi sen 1/1 -> Sum1/3
  Sum1/1 -> Sum7/1
  Sum/1 -> Sum4/1
  Constant/1 -> Sum/1
  pos Sen 4/1 -> Sum2/2
  pos Sen 2/1 -> Sum2/1
  pos Sen 3/1 -> Sum2/3
  Sum2/1 -> Sum3/1
  pos Sen 5/1 -> Sum3/2
  Sum3/1 -> Sum4/2
  Sum4/1 -> desired position/1
  psi sen 3/1 -> Sum5/2
  Sum5/1 -> Sum6/1
  Sum6/1 -> Sum7/2
  psi sen 5/1 -> Sum6/2
  psi sen 4/1 -> Sum5/3
  psi sen 2/1 -> Sum5/1
  Sum7/1 -> Selector/1
  Constant1/1 -> Sum1/1
  Selector/1 -> desired Heading/1

== system Aearial_Inspection_UAV_Simulation/Path Palnner/Arm Guid/Manual ==
  Enable : EnablePort
  Chart : Stateflow chart  TreatAsAtomicUnit=on
      settings: PortSchema="{\"entries\":[{\"content\":{\"sides\":[{\"content\":{\"connectorIds\":[\"In2\"]},\"type\":\"ConnectorPlacement.EquallySpacedRectSide\",\"uuid\":\"d41aa2ef-851b-45b8-8e6c-1053e1d243b7\"},{\"content\":{\"connectorIds\":[\"Out1\",\"Out2\",\"Out3\",\"Out4\"],\"side\":\"RIGHT\"},\"type\":\"ConnectorPlacement.EquallySpacedRectSide\",\"uuid\":\"08118517-e11e-47f6-b3dd-e648183d48c6\"},{\"content\":{\"connectorIds\":[],\"side\":\"TOP\"},\"type\":\"ConnectorPlacement.EquallySpacedRectSide\",\"uuid\":\"01724f1f-a9bc-4e8d-98b3-a6ae72a7ff1d\"},{\"content\":{\"connectorIds\":[\"In1\"],\"side\":\"BOTTOM\"},\"type\":\"ConnectorPlacement.EquallySpacedRectSide\",\"uuid\":\"10ef03df-cc44-462b-b183-21fd4d15a238\"}]},\"type\":\"ConnectorPlacement.EquallySpacedConnector\",\"uuid\":\"e78f7f87-3af7-476c-b648-97c17ec8585e\"}],\"packageUris\":[\"http://schema.mathworks.com/mf0/Connector/R2020b\"],\"version\":\"1.0\"}"
  Keyboard 1 : M-S-Function  FunctionName=sfun_keyboard_input_v1_2b  mask(Keyboard Input){}
      mask help: Keyboard Input
      mask Display: fprintf('Keyboard');
  Mux7 : Mux  Inputs=2
  Mux8 : Mux  Inputs=2
  desired position : Outport  PortDimensions=3
  desired Heading : Outport  Port=2  PortDimensions=1
  wires:
  Keyboard 1/2 -> Chart/1(hit)
  Mux8/1 -> Mux7/1
  Keyboard 1/1 -> Chart/2(key)
  Mux7/1 -> desired position/1
  Chart/1(xd) -> Mux8/1
  Chart/3(zd) -> Mux7/2
  Chart/2(yd) -> Mux8/2
  Chart/4(sd) -> desired Heading/1  "desired Heading"

== system Aearial_Inspection_UAV_Simulation/Path Palnner/Arm Guid/Senario 1 ==
  Enable : EnablePort
  Clock : Clock
  senario_1 : MATLAB Function  TreatAsAtomicUnit=on
  desired position : Outport  PortDimensions=3
  desired Heading : Outport  Port=2  PortDimensions=1
  wires:
  senario_1/1(desired_pos) -> desired position/1
  senario_1/2(desired_psi) -> desired Heading/1
  Clock/1 -> senario_1/1(t)

== system Aearial_Inspection_UAV_Simulation/Path Palnner/Arm Guid/Senario 2 ==
  Enable : EnablePort
  Clock : Clock
  senario_2 : MATLAB Function  TreatAsAtomicUnit=on
  desired position : Outport  PortDimensions=3
  desired Heading : Outport  Port=2
  wires:
  Clock/1 -> senario_2/1(t)
  senario_2/2(desired_psi) -> desired Heading/1
  senario_2/1(desired_pos) -> desired position/1
